simulink model "simMalhaFechadaGanhoProporcionalRetornoUnitario"  (R2019b)
settings: Solver=VariableStepAuto  StartTime=0.0  StopTime=10.0  MaxStep=0.01  RelTol=1e-3
undefined symbols (not defined in the file or in its folder): k
settings Model: Creator=feliperocha  LastModifiedBy=feliperocha

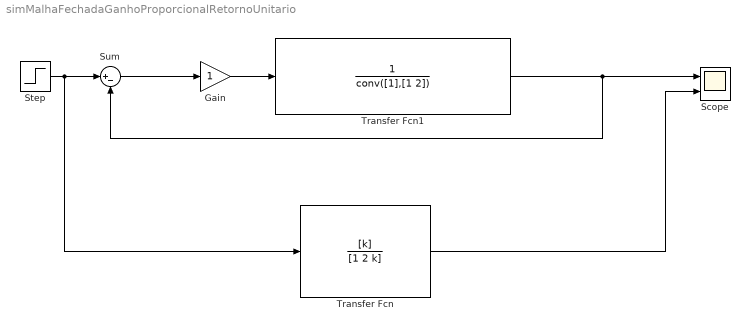
== system simMalhaFechadaGanhoProporcionalRetornoUnitario ==
  Gain : Gain
  Scope : Scope  NumInputPorts=2
  Step : Step  SampleTime=0
  Sum : Sum  Inputs=|+-
  Transfer Fcn : TransferFcn  Numerator=[k]  Denominator=[1 2 k]
  Transfer Fcn1 : TransferFcn  Denominator=conv([1],[1 2])
  wires:
  Transfer Fcn/1 -> Scope/2
  Transfer Fcn1/1 -> Sum/2, Scope/1
  Step/1 -> Transfer Fcn/1, Sum/1
  Sum/1 -> Gain/1
  Gain/1 -> Transfer Fcn1/1
